simulink model "model_2024b_version"  (R2024b)
settings: Solver=ode4  StartTime=0.0  StopTime=80  FixedStep=Sample_Time  RelTol=1e-3
InitFcn:
  | addpath(genpath(fileparts(which(bdroot))));
  | [cspar, ccpar, ckpar] = s_params();
model workspace: external: MATLAB File model_2024b_version_saveas.m (data not in the file)
undefined symbols (not defined in the file or in its folder): Sample_Time
settings Model: SimulationMode=accelerator  Creator=loren  LastModifiedBy=loren
settings RTWCC: GPUComputeCapability=3.5
settings GRTTargetCC: RTWCAPISignals=on  RTWCAPIParams=on

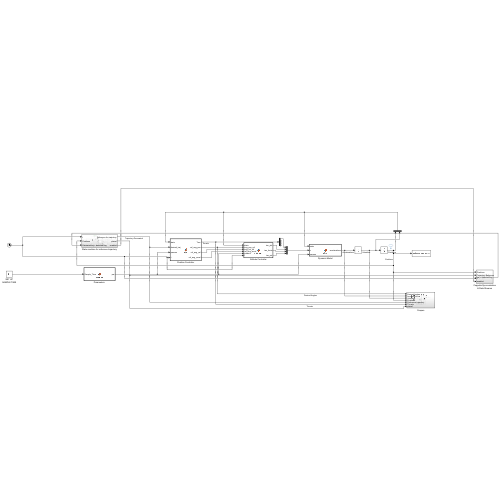
[thumbnail: Simulink's stored preview of the top-level diagram]
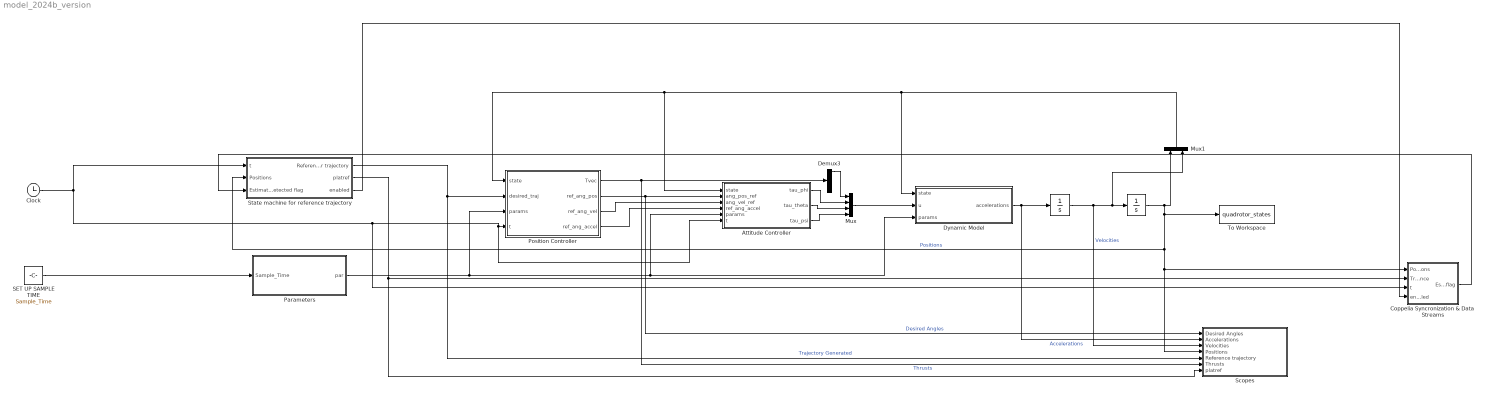
== system model_2024b_version ==
  " " : Integrator  InitialCondition=[0 0 0 0 0 0]
  "  " : Integrator  InitialCondition=[0 0 0 0 0 0]
  Attitude Controller : MATLAB Function  TreatAsAtomicUnit=on  SystemSampleTime=Sample_Time
  Clock : Clock
  Coppelia Syncronization & Data Streams : Subsystem
  Demux3 : Demux
  Dynamic Model : MATLAB Function  TreatAsAtomicUnit=on
  Mux : Mux
  Mux1 : Mux  Inputs=2
  "Parameters " : MATLAB Function  TreatAsAtomicUnit=on  SystemSampleTime=Sample_Time
  Position Controller : MATLAB Function  TreatAsAtomicUnit=on  SystemSampleTime=Sample_Time
  SET UP SAMPLE TIME : Constant  Value=Sample_Time
  Scopes : Subsystem
  State machine for reference trajectory : Subsystem
  To Workspace : ToWorkspace  VariableName=quadrotor_states  SaveFormat=Structure With Time  SampleTime=-1
  wires:
  "Parameters "/1(par) -> Dynamic Model/3(params), Attitude Controller/5(params), Position Controller/3(params)
  Position Controller/2(ref_ang_pos) -> Scopes/1(Desired Angles), Attitude Controller/2(ang_pos_ref)  "Desired Angles"
  Position Controller/3(ref_ang_vel) -> Attitude Controller/3(ang_vel_ref)
  Attitude Controller/1(tau_phi) -> Mux/2
  Attitude Controller/2(tau_theta) -> Mux/3
  Attitude Controller/3(tau_psi) -> Mux/4
  Mux/1 -> Dynamic Model/2(u)
  Dynamic Model/1(accelerations) -> " "/1, Scopes/2(Accelerations)  "Accelerations"
  " "/1 -> "  "/1, Mux1/2, Scopes/3(Velocities)  "Velocities"
  Mux1/1 -> Dynamic Model/1(state), Position Controller/1(state), Attitude Controller/1(state)
  Clock/1 -> Attitude Controller/6(t), Position Controller/4(t), Coppelia Syncronization & Data Streams/3(t), State machine for reference trajectory/1(t)
  "  "/1 -> State machine for reference trajectory/2(Positions), Scopes/4(Positions), Coppelia Syncronization & Data Streams/1(Positions), To Workspace/1, Mux1/1  "Positions"
  SET UP SAMPLE TIME/1 -> "Parameters "/1(Sample_Time)
  Demux3/1 -> Mux/1
  State machine for reference trajectory/1(Reference for trajectory) -> Scopes/5(Reference trajectory), Position Controller/2(desired_traj)  "Trajectory Generated"
  Position Controller/4(ref_ang_accel) -> Attitude Controller/4(ref_ang_accel)
  State machine for reference trajectory/2(platref) -> Scopes/7(platref), Coppelia Syncronization & Data Streams/2(Trajectory Reference)
  Position Controller/1(Tvec) -> Demux3/1, Scopes/6(Thrusts)  "Thrusts"
  Coppelia Syncronization & Data Streams/1(Estimated traj + detected flag) -> State machine for reference trajectory/3(Estimated traj + detected flag)
  State machine for reference trajectory/3(enabled) -> Coppelia Syncronization & Data Streams/4(enabled)

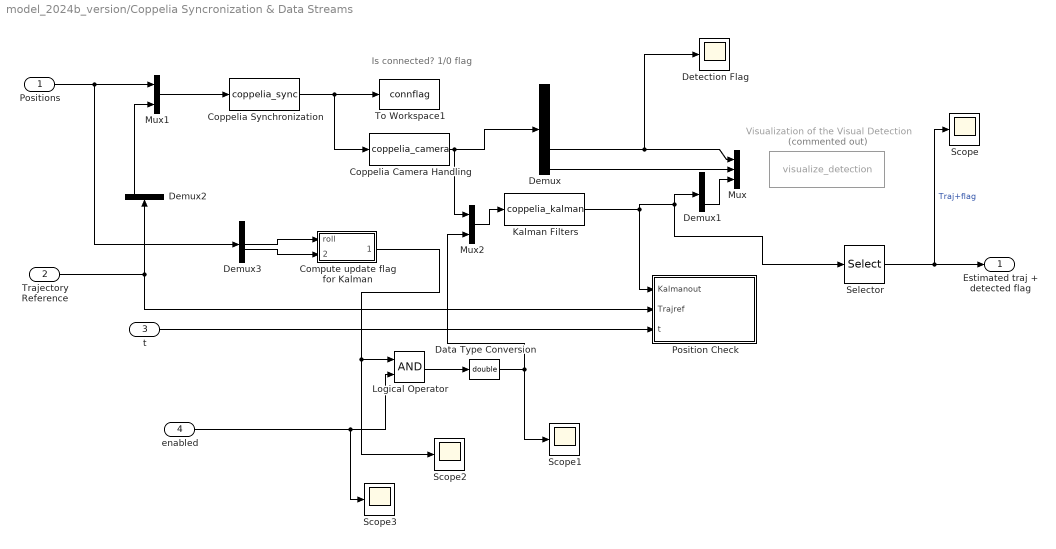
== system model_2024b_version/Coppelia Syncronization & Data Streams ==
  note: Is connected? 1/0 flag
  Positions : Inport
  Trajectory Reference : Inport  Port=2
  t : Inport  Port=3
  enabled : Inport  Port=4
  Compute update flag for Kalman : MATLAB Function  TreatAsAtomicUnit=on  SystemSampleTime=Sample_Time
  Coppelia Camera Handling : S-Function  Priority=1  FunctionName=coppelia_camera  Parameters=ccpar  SFunctionDeploymentMode=off  EnableBusSupport=off
  Coppelia Synchronization : S-Function  Priority=-1  FunctionName=coppelia_sync  Parameters=cspar  SFunctionDeploymentMode=off  EnableBusSupport=off
  Data Type Conversion : DataTypeConversion  OutDataTypeStr=double  SaturateOnIntegerOverflow=off  RndMeth=Floor
  Demux : Demux  Outputs=5
  Demux1 : Demux  Outputs=8
  Demux2 : Demux  Outputs=2
  Demux3 : Demux  Outputs=6
  Detection Flag : Scope
  Kalman Filters : S-Function  Priority=1  FunctionName=coppelia_kalman  Parameters=ckpar  SFunctionDeploymentMode=off  EnableBusSupport=off
  Logical Operator : Logic  AllPortsSameDT=off  OutDataTypeStr=boolean
  Mux : Mux  Inputs=3
  Mux1 : Mux  Inputs=2
  Mux2 : Mux  Inputs=2
  Position Check : MATLAB Function  TreatAsAtomicUnit=on  SystemSampleTime=Sample_Time
  Scope{,1..3} (4 alike) : Scope
  Selector : Selector  InputPortWidth=8  IndexOptions=Index vector (dialog)  Indices=1:7  OutputSizes=1
  To Workspace1 : ToWorkspace  VariableName=connflag  SaveFormat=Timeseries  SampleTime=-1
  Visualization of the Visual Detection : S-Function  Commented=on  FunctionName=visualize_detection  SFunctionDeploymentMode=off  EnableBusSupport=off
  Estimated traj + detected flag : Outport
  wires:
  Coppelia Synchronization/1 -> To Workspace1/1, Coppelia Camera Handling/1
  Positions/1 -> Demux3/1, Mux1/1
  Kalman Filters/1 -> Position Check/1(Kalmanout), Demux1/1, Selector/1
  Coppelia Camera Handling/1 -> Mux2/1, Demux/1
  Demux/4 -> Detection Flag/1, Mux/1
  Demux/5 -> Mux/2
  Trajectory Reference/1 -> Position Check/2(Trajref), Demux2/1
  t/1 -> Position Check/3(t)
  Mux1/1 -> Coppelia Synchronization/1
  Demux2/1 -> Mux1/2
  Selector/1 -> Scope/1, Estimated traj + detected flag/1  "Traj+flag"
  Demux3/4 -> Compute update flag for Kalman/1(roll)
  Demux3/5 -> Compute update flag for Kalman/2(pitch)
  Mux2/1 -> Kalman Filters/1
  enabled/1 -> Scope3/1, Logical Operator/2
  Demux1/7 -> Mux/3
  Compute update flag for Kalman/1(enable_update) -> Scope2/1, Logical Operator/1
  Logical Operator/1 -> Data Type Conversion/1
  Data Type Conversion/1 -> Mux2/2, Scope1/1

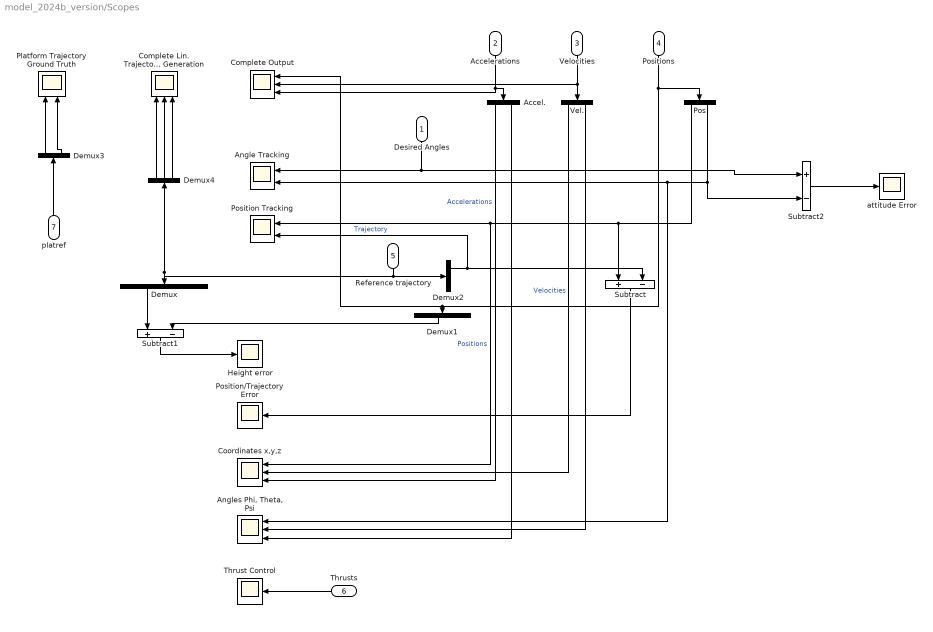
== system model_2024b_version/Scopes ==
  Desired Angles : Inport
  Accelerations : Inport  Port=2
  Velocities : Inport  Port=3
  Positions : Inport  Port=4
  Reference trajectory : Inport  Port=5
  Thrusts : Inport  Port=6
  platref : Inport  Port=7
  Accel. : Demux  Tag=Accelerations  Outputs=2
  Angle Tracking : Scope  NumInputPorts=2
  "Angles Phi, Theta, Psi" : Scope  NumInputPorts=3
  Complete Lin. Trajectory Generation : Scope  NumInputPorts=3
  Complete Output : Scope  NumInputPorts=3
  Coordinates x,y,z : Scope  NumInputPorts=3
  Demux : Demux  Outputs=9
  Demux1 : Demux  Outputs=6
  Demux2 : Demux  Outputs=3
  Demux3 : Demux  Outputs=2
  Demux4 : Demux  Outputs=3
  Height error : Scope
  Platform Trajectory Ground Truth : Scope  NumInputPorts=2
  Pos : Demux  Outputs=2
  Position Tracking : Scope  NumInputPorts=2
  Position/Trajectory Error : Scope
  Subtract : Sum  Inputs=+-
  Subtract1 : Sum  Inputs=+-
  Subtract2 : Sum  Inputs=+-
  Thrust Control : Scope
  Vel. : Demux  Outputs=2
  attitude Error : Scope
  wires:
  Accel./1 -> Coordinates x,y,z/3  "Accelerations"
  Pos/2 -> Subtract2/2, "Angles Phi, Theta, Psi"/1, Angle Tracking/2
  Accelerations/1 -> Complete Output/3, Accel./1
  Accel./2 -> "Angles Phi, Theta, Psi"/3
  Vel./2 -> "Angles Phi, Theta, Psi"/2
  Velocities/1 -> Vel./1, Complete Output/2
  Positions/1 -> Pos/1, Complete Output/1, Demux1/1
  Pos/1 -> Position Tracking/1, Coordinates x,y,z/1, Subtract/1  "Positions"
  Vel./1 -> Coordinates x,y,z/2  "Velocities"
  Desired Angles/1 -> Angle Tracking/1, Subtract2/1
  Subtract/1 -> Position/Trajectory Error/1
  Demux2/1 -> Position Tracking/2, Subtract/2  "Trajectory"
  Reference trajectory/1 -> Demux4/1, Demux/1, Demux2/1
  Demux4/2 -> Complete Lin. Trajectory Generation/2
  Demux4/3 -> Complete Lin. Trajectory Generation/3
  Demux4/1 -> Complete Lin. Trajectory Generation/1
  Demux/3 -> Subtract1/1
  Demux1/3 -> Subtract1/2
  Subtract1/1 -> Height error/1
  Thrusts/1 -> Thrust Control/1
  platref/1 -> Demux3/1
  Demux3/2 -> Platform Trajectory Ground Truth/2
  Demux3/1 -> Platform Trajectory Ground Truth/1
  Subtract2/1 -> attitude Error/1

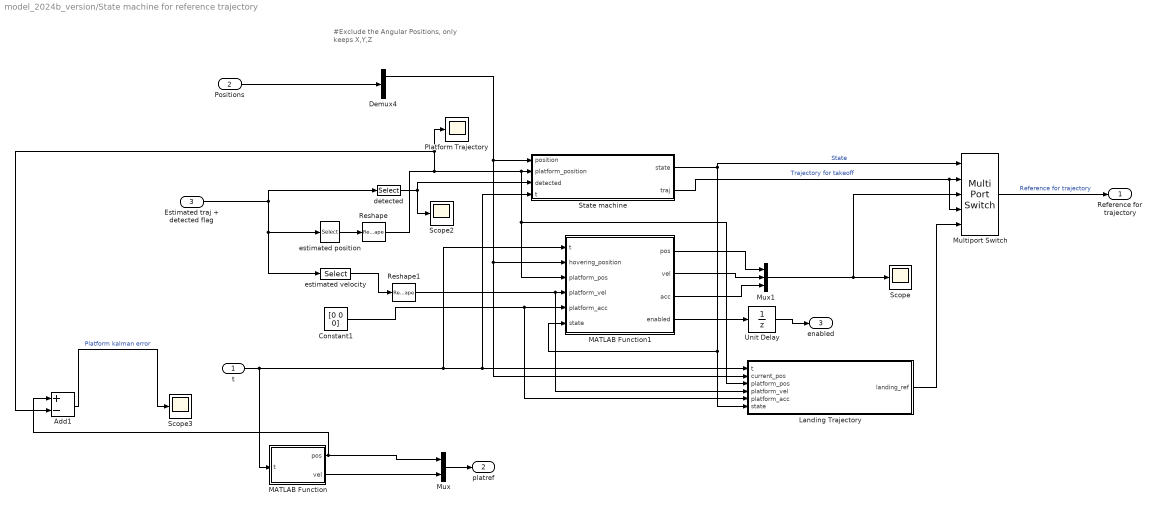
== system model_2024b_version/State machine for reference trajectory ==
  note: #Exclude the Angular Positions,
      | only keeps X,Y,Z
  t : Inport
  Positions : Inport  Port=2
  Estimated traj + detected flag : Inport  Port=3
  Add1 : Sum  Inputs=+-
  Constant1 : Constant  Value=[0 0 0]
  Demux4 : Demux  Outputs=2
  Landing Trajectory : MATLAB Function  TreatAsAtomicUnit=on  SystemSampleTime=Sample_Time
  MATLAB Function : MATLAB Function  TreatAsAtomicUnit=on
  MATLAB Function1 : MATLAB Function  TreatAsAtomicUnit=on  SystemSampleTime=Sample_Time
  Multiport Switch : MultiPortSwitch  Inputs=4  SaturateOnIntegerOverflow=off  InputSameDT=off
  Mux : Mux  Inputs=2
  Mux1 : Mux  Inputs=3
  Platform Trajectory : Scope
  Reshape : Reshape  OutputDimensionality=Row vector (2-D)
  Reshape1 : Reshape  OutputDimensionality=Row vector (2-D)
  Scope : Scope
  Scope2 : Scope
  Scope3 : Scope
  State machine : MATLAB Function  TreatAsAtomicUnit=on  SystemSampleTime=Sample_Time
  Unit Delay : UnitDelay  SampleTime=Sample_Time  HasFrameUpgradeWarning=on
  detected : Selector  InputPortWidth=7  IndexOptions=Index vector (dialog)  Indices=[7]  OutputSizes=1
  estimated position : Selector  InputPortWidth=7  IndexOptions=Index vector (dialog)  Indices=[1 2 3]  OutputSizes=1
  estimated velocity : Selector  InputPortWidth=7  IndexOptions=Index vector (dialog)  Indices=4:6  OutputSizes=1
  Reference for trajectory : Outport
  platref : Outport  Port=2
  enabled : Outport  Port=3
  wires:
  State machine/1(state) -> Multiport Switch/1, MATLAB Function1/6(state), Landing Trajectory/6(state)  "State"
  estimated position/1 -> Reshape/1
  t/1 -> MATLAB Function/1(t), MATLAB Function1/1(t), State machine/4(t), Landing Trajectory/1(t)
  Demux4/1 -> Landing Trajectory/2(current_pos), MATLAB Function1/2(hovering_position), State machine/1(position)
  Multiport Switch/1 -> Reference for trajectory/1  "Reference for trajectory"
  Positions/1 -> Demux4/1
  Landing Trajectory/1(landing_ref) -> Multiport Switch/5
  State machine/2(traj) -> Multiport Switch/4, Multiport Switch/2  "Trajectory for takeoff"
  Mux/1 -> platref/1
  Estimated traj + detected flag/1 -> estimated velocity/1, estimated position/1, detected/1
  detected/1 -> Scope2/1, State machine/3(detected)
  MATLAB Function/1(pos) -> Add1/1, Mux/1
  MATLAB Function/2(vel) -> Mux/2
  MATLAB Function1/1(pos) -> Mux1/1
  MATLAB Function1/2(vel) -> Mux1/2
  MATLAB Function1/3(acc) -> Mux1/3
  Mux1/1 -> Scope/1, Multiport Switch/3
  MATLAB Function1/4(enabled) -> Unit Delay/1
  Unit Delay/1 -> enabled/1
  Constant1/1 -> MATLAB Function1/5(platform_acc), Landing Trajectory/5(platform_acc)
  Reshape/1 -> Add1/2, Platform Trajectory/1, MATLAB Function1/3(platform_pos), Landing Trajectory/3(platform_pos), State machine/2(platform_position)
  Reshape1/1 -> Landing Trajectory/4(platform_vel), MATLAB Function1/4(platform_vel)
  estimated velocity/1 -> Reshape1/1
  Add1/1 -> Scope3/1  "Platform kalman error"

== matlab function model_2024b_version/State machine for reference trajectory/Landing Trajectory ==
  data: t input; landing_ref output size=[1 9]; current_pos input size=[1 3]; platform_pos input; platform_vel input; platform_acc input; state input
function landing_ref = landing_trajectory(t, current_pos, platform_pos, platform_vel, platform_acc, state)

[pos, vel, acc] = landing_trajectory(t, current_pos, platform_pos, platform_vel, platform_acc, state);
landing_ref = [pos, vel, acc];

== matlab function model_2024b_version/Coppelia Syncronization & Data Streams/Compute update flag for Kalman ==
  data: roll input; enable_update output; pitch input
function enable_update = compute_kalman_update_flag(roll, pitch)

enable_update = compute_kalman_update_flag(roll, pitch);

== matlab function model_2024b_version/State machine for reference trajectory/MATLAB Function1 ==
  data: t input; pos output; hovering_position input; platform_pos input; platform_vel input; platform_acc input; state input; vel output; acc output; enabled output
function [pos, vel, acc, enabled] = smooth_start_tracking(t, hovering_position, platform_pos, platform_vel, platform_acc, state)

[pos, vel, acc, enabled] = smooth_start_tracking(t, hovering_position, platform_pos, platform_vel, platform_acc, state);

== matlab function model_2024b_version/Position Controller ==
  data: Tvec output; state input; desired_traj input; ref_ang_pos output; ref_ang_vel output; params input; t input; ref_ang_accel output
function [Tvec,ref_ang_pos,ref_ang_vel, ref_ang_accel] = pos(state,desired_traj,params,t)

[Tvec,ref_ang_pos,ref_ang_vel, ref_ang_accel] = position_control(desired_traj,state,params);

== matlab function model_2024b_version/Parameters  ==
  data: par output; Sample_Time input
function par = params(Sample_Time)

[m,g,Ix,Iy,Iz,Kp_pos,Kd_pos,Ki_pos,Kp_ang,Kd_ang,Ki_ang,dt] = model_n_control_param();
%overwrites the Sample Time with the Environment sample time
dt=Sample_Time;
par = [m,g,Ix,Iy,Iz,Kp_pos,Kd_pos,Ki_pos,Kp_ang,Kd_ang,Ki_ang,dt];

== matlab function model_2024b_version/Attitude Controller ==
  data: state input; ang_pos_ref input; tau_phi output size=1; ang_vel_ref input; ref_ang_accel input; params input; tau_theta output size=1; tau_psi output size=1; t input
function [tau_phi,tau_theta,tau_psi] = attitude(state,ang_pos_ref,ang_vel_ref,ref_ang_accel,params,t)

[tau_phi,tau_theta,tau_psi] = attitude_control(ang_pos_ref,ang_vel_ref,ref_ang_accel,state,params);

== matlab function model_2024b_version/Dynamic Model ==
  data: state input; u input; accelerations output; params input
function accelerations = dyn(state,u,params)

accelerations = dynamic_model(state, u, params);

== matlab function model_2024b_version/State machine for reference trajectory/State machine ==
  data: position input; platform_position input; detected input; t input; state output; traj output size=[1 9]
function [state, traj]  = state_manager(position,platform_position, detected, t)

[state, traj] = stateManager(position,platform_position, detected, t);

== matlab function model_2024b_version/Coppelia Syncronization & Data Streams/Position Check ==
  data: Kalmanout input; Trajref input; t input
function fcn(Kalmanout, Trajref, t)

detected = Kalmanout(7);
initialized = Kalmanout(8);

if initialized && detected && mod(t, 0.1) == 0
    fprintf('  [REAL POSITION] pos=[%.3f, %.3f, %.3f], vel=[%.3f, %.3f, %.3f]\n', ...
        Trajref(1), Trajref(2), Trajref(3), Trajref(4), Trajref(5), Trajref(6));
end

end

== matlab function model_2024b_version/State machine for reference trajectory/MATLAB Function ==
  data: t input; pos output; vel output
function [pos,vel] = platform_trajectory(t)

[pos, vel] = platform_trajectory(t);
